simulink model "TGB_V0001"  (R2016b)
settings: Solver=VariableStepAuto  StartTime=0.0  StopTime=350  RelTol=1e-3
values from neighbouring files (symbols this model uses):
  AntiW = 2    [AutoPID.m]
  CIPD = 2    [AutoPID.m]
  Dev = 2    [AutoPID.m]
  h = 30    [AutoPID.m]
  K = data.Data(len)/100    [AutoPID.m]
  Kp = 0.6*Kc    (= 0.48762365543)    [AutoPID.m]
  Malha = 1    [AutoPID.m]
  T = (100*wn)/2*pi    [AutoPID.m]
  tau = (3/2)*(t2-t1)    [AutoPID.m]
  Td = Tc*0.125    (= 41.8060200669)    [AutoPID.m]
  theta = t2-tau    [AutoPID.m]
  Ti = Tc*0.5    (= 167.224080268)    [AutoPID.m]
  TypeController = 1    [AutoPID.m]
  TypeOutput = 1    [AutoPID.m]
undefined symbols (not defined in the file or in its folder): DiscIntNeverNeededParam
libraries: simulink x2
settings Model: Creator=Workstation - LFC  LastModifiedBy=Gpiaia
settings DataIOCC: SaveOutput=off  SaveTime=off
settings OptimizationCC: DefaultParameterBehavior=Inlined  UseDivisionForNetSlopeComputation=on  UseFloatMulNetSlope=on  InlineInvariantSignals=on  PassReuseOutputArgsAs=Individual arguments  ZeroExternalMemoryAtStartup=off  ZeroInternalMemoryAtStartup=off  NoFixptDivByZeroProtection=on  EfficientFloat2IntCast=on  LifeSpan=1
settings DebuggingCC: ParameterTunabilityLossMsg=error  SFExecutionAtInitializationDiag=none
settings HardwareCC: ProdBitPerLong=64  ProdHWDeviceType=Intel->x86-64 (Linux 64)
settings RTWCC: SystemTargetFile=ert.tlc  TemplateMakefile=ert_default_tmf  Description=Embedded Coder  GenerateReport=on  IncludeHyperlinkInReport=on  LaunchReport=on  GenerateTraceInfo=on  GenerateTraceReport=on  GenerateTraceReportSl=on  GenerateTraceReportSf=on  GenerateTraceReportEml=on  GenerateCodeMetricsReport=on
settings CodeAppCC: ForceParamTrailComments=on  IgnoreCustomStorageClasses=off  OperatorAnnotations=on  SimulinkDataObjDesc=on  SFDataObjDesc=on  MATLABFcnDesc=on  CustomSymbolStrGlobalVar=rt$N$M  CustomSymbolStrType=$N$M  CustomSymbolStrFcn=$N$M$F  CustomSymbolStrMacro=$N$M  InsertBlockDesc=on  MATLABSourceComments=on
settings ERTTargetCC: TargetLangStandard=C99 (ISO)  GenerateSampleERTMain=on  CombineSignalStateStructs=on  SupportComplex=off  SupportNonInlinedSFcns=on  InlinedParameterPlacement=NonHierarchical  ERTCustomFileTemplate=example_file_process.tlc  ERTFilePackagingFormat=CompactWithDataFile

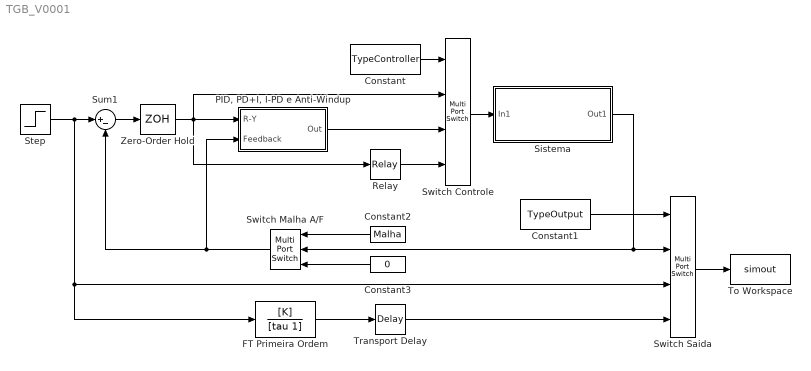
== system TGB_V0001 ==
  Constant : Constant  Value=TypeController
  Constant1 : Constant  Value=TypeOutput
  Constant2 : Constant  Value=Malha
  Constant3 : Constant  Value=0
  FT Primeira Ordem : TransferFcn  Numerator=[K]  Denominator=[tau 1]
  "PID, PD+I, I-PD e Anti-Windup" : Subsystem
  Relay : Relay  OnSwitchValue=+h  OffSwitchValue=-h  OnOutputValue=+h  OffOutputValue=-h
  Sistema : Subsystem
      mask help: Simulink:masks:GenSFuncDesc_MD
      mask Help: eval('feval(''rtwprivate'',''rtwhelpview'',''rtw_sfcn_block'')');
  Step : Step  Time=0  After=100  SampleTime=0
  Sum1 : Sum  Inputs=|+-
  Switch Controle : MultiPortSwitch  SaturateOnIntegerOverflow=on
  Switch Malha A/F : MultiPortSwitch  Inputs=2  SaturateOnIntegerOverflow=on
  Switch Saida : MultiPortSwitch  SaturateOnIntegerOverflow=on
  To Workspace : ToWorkspace  VariableName=simout  SaveFormat=Timeseries  SampleTime=-1
  Transport Delay : TransportDelay  DelayTime=theta
  Zero-Order Hold : ZeroOrderHold  SampleTime=T
  wires:
  Sum1/1 -> Zero-Order Hold/1
  Step/1 -> FT Primeira Ordem/1, Switch Saida/3, Sum1/1
  FT Primeira Ordem/1 -> Transport Delay/1
  Sistema/1(Out1) -> Switch Saida/2, Switch Malha A/F/2
  Zero-Order Hold/1 -> "PID, PD+I, I-PD e Anti-Windup"/1(R-Y), Switch Controle/2, Relay/1
  Transport Delay/1 -> Switch Saida/4
  Switch Saida/1 -> To Workspace/1
  Constant/1 -> Switch Controle/1
  Constant1/1 -> Switch Saida/1
  Switch Malha A/F/1 -> "PID, PD+I, I-PD e Anti-Windup"/2(Feedback), Sum1/2
  Constant2/1 -> Switch Malha A/F/1
  Constant3/1 -> Switch Malha A/F/3
  Switch Controle/1 -> Sistema/1(In1)
  "PID, PD+I, I-PD e Anti-Windup"/1(Out) -> Switch Controle/3
  Relay/1 -> Switch Controle/4

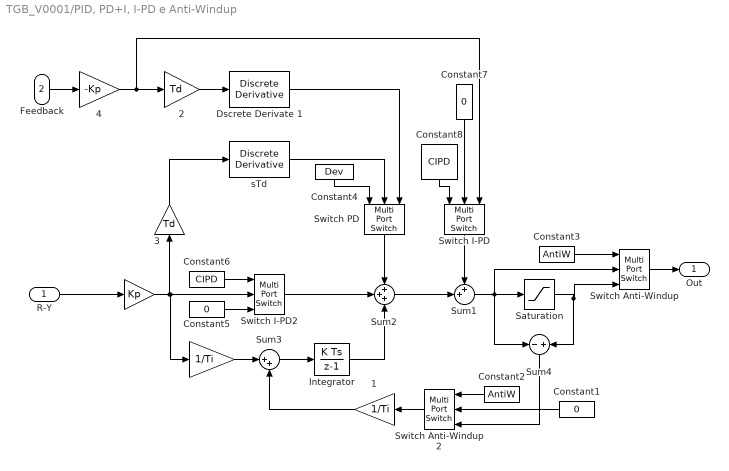
== system TGB_V0001/PID, PD+I, I-PD e Anti-Windup ==
  R-Y : Inport
  Feedback : Inport  Port=2
  " " : Gain  Gain=Kp
  " 3" : Gain  Gain=Td
  "  " : Gain  Gain=1/Ti
  "  1" : Gain  Gain=1/Ti
  "  2" : Gain  Gain=Td
  "  4" : Gain  Gain=-Kp
  Constant1 : Constant  Value=0
  Constant2 : Constant  Value=AntiW
  Constant3 : Constant  Value=AntiW
  Constant4 : Constant  Value=Dev
  Constant5 : Constant  Value=0
  Constant6 : Constant  Value=CIPD
  Constant7 : Constant  Value=0
  Constant8 : Constant  Value=CIPD
  Dscrete Derivate 1 : simulink/Discrete/Discrete Derivative  gainval=1  ICPrevScaledInput=0.0  OutMin=[]  OutMax=[]  OutDataType=fixdt(1, 16)  OutScaling=2^-10  DoSatur=off
  Integrator : DiscreteIntegrator  gainval=1  InitialConditionSetting=State (most efficient)  SampleTime=T  ICPrevOutput=DiscIntNeverNeededParam  ICPrevScaledInput=DiscIntNeverNeededParam
  Saturation : Saturate  UpperLimit=90  LowerLimit=-90
  Sum1 : Sum  Inputs=++|
  Sum2 : Sum  Inputs=+++
  Sum3 : Sum  Inputs=|++
  Sum4 : Sum  Inputs=-+
  Switch Anti-Windup : MultiPortSwitch  Inputs=2  SaturateOnIntegerOverflow=on
  Switch Anti-Windup 2 : MultiPortSwitch  Inputs=2  SaturateOnIntegerOverflow=on
  Switch I-PD : MultiPortSwitch  Inputs=2  SaturateOnIntegerOverflow=on
  Switch I-PD2 : MultiPortSwitch  Inputs=2  SaturateOnIntegerOverflow=on
  Switch PD : MultiPortSwitch  Inputs=2  SaturateOnIntegerOverflow=on
  sTd : simulink/Discrete/Discrete Derivative  gainval=1  ICPrevScaledInput=0.0  OutMin=[]  OutMax=[]  OutDataType=fixdt(1, 16)  OutScaling=2^-10  DoSatur=off
  Out : Outport
  wires:
  Integrator/1 -> Sum2/3
  Sum3/1 -> Integrator/1
  "  1"/1 -> Sum3/2
  "  "/1 -> Sum3/1
  Saturation/1 -> Switch Anti-Windup/3, Sum4/2
  "  2"/1 -> Dscrete Derivate 1/1
  Switch Anti-Windup/1 -> Out/1
  Switch Anti-Windup 2/1 -> "  1"/1
  Constant2/1 -> Switch Anti-Windup 2/1
  Constant3/1 -> Switch Anti-Windup/1
  Switch PD/1 -> Sum2/1
  Dscrete Derivate 1/1 -> Switch PD/3
  Constant4/1 -> Switch PD/1
  " 3"/1 -> sTd/1
  sTd/1 -> Switch PD/2
  R-Y/1 -> " "/1
  " "/1 -> Switch I-PD2/2, "  "/1, " 3"/1
  Switch I-PD2/1 -> Sum2/2
  Constant5/1 -> Switch I-PD2/3
  Constant6/1 -> Switch I-PD2/1
  Feedback/1 -> "  4"/1
  "  4"/1 -> Switch I-PD/3, "  2"/1
  Sum2/1 -> Sum1/2
  Sum1/1 -> Switch Anti-Windup/2, Sum4/1, Saturation/1
  Constant8/1 -> Switch I-PD/1
  Switch I-PD/1 -> Sum1/1
  Constant7/1 -> Switch I-PD/2
  Constant1/1 -> Switch Anti-Windup 2/2
  Sum4/1 -> Switch Anti-Windup 2/3

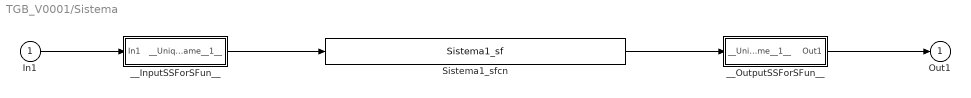
== system TGB_V0001/Sistema ==
  In1 : Inport
  Sistema1_sfcn : S-Function  FunctionName=Sistema1_sf  SFunctionModules=""  SFunctionDeploymentMode=off  EnableBusSupport=off  mask{rtw_sf_name=Sistema1_sf, showVar=off}
      mask prompts: rtw_sf_name "Simulink:masks:GenSFuncName_MP"; showVar "Simulink:masks:GenSFuncShowModuleList_MP"
      mask help: Simulink:masks:GenSFuncDesc_MD
      mask init:
      | displist = '';
      | if ~strcmp(get_param(gcb, 'FunctionName'), rtw_sf_name);
      |   set_param(gcb, 'FunctionName', rtw_sf_name);
      | end
      | % Check if we are generating code
      | rtw_mode = false;
      | if strcmpi(get_param(bdroot(gcb),'SimulationStatus'),'Initializing')
      | 	rtw_mode = strcmpi(get_param(bdroot(gcb),'BuildingRTWCode'),'on') && ...
      | 		~strcmpi(get_param(bdroot(gcb),'TargetStyle'),'SimulationTarget');
      | end
      | if showVar || rtw_mode
      | 	if exist('rtwsfunc') == 2 | exist('rtwsfunc') == 6
      | 		tmplist = rtwsfunc(rtw_sf_name,gcb);
      | 		tmplist = DAStudio.message('Simulink:masks:GenSFuncListOfModules_IC', tmplist);
      | 	elseif showVar
      | 		tmplist1 = DAStudio.message('Simulink:masks:GenSFuncListOfModules_IC', '');
      |         tmplist2 = DAStudio.message('Simulink:masks:GenSFuncNotLicensed_IC');
      |         tmplist = [tmplist1 tmplist2];
      |  	end
      | end
      | if showVar
      |   displist = tmplist;
      | end
      settings: CopyFcn=|
      | if ~strcmp(get_param(gcb,'Linkstatus'),'none') && ...
      | ~strcmp(get_param(gcb,'Linkstatus'),'implicit')
      |   set_param(gcb,'LinkStatus','none');
      | end
      mask Help: eval('feval(''rtwprivate'',''rtwhelpview'',''rtw_sfcn_block'')');
      mask Display:
      | port_label('input',1,'In1');
      | port_label('output',1,'Out1');
  __InputSSForSFun__ : Subsystem
  __OutputSSForSFun__ : Subsystem
  Out1 : Outport
  wires:
  In1/1 -> __InputSSForSFun__/1(In1)
  __InputSSForSFun__/1(__UniqueOutportName__1__) -> Sistema1_sfcn/1
  Sistema1_sfcn/1 -> __OutputSSForSFun__/1(__UniqueInportName__1__)
  __OutputSSForSFun__/1(Out1) -> Out1/1

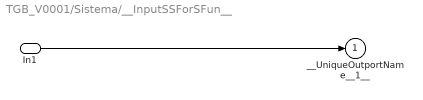
== system TGB_V0001/Sistema/__InputSSForSFun__ ==
  In1 : Inport
  __UniqueOutportName__1__ : Outport
  wires:
  In1/1 -> __UniqueOutportName__1__/1

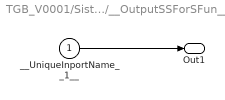
== system TGB_V0001/Sistema/__OutputSSForSFun__ ==
  __UniqueInportName__1__ : Inport
  Out1 : Outport
  wires:
  __UniqueInportName__1__/1 -> Out1/1
